simulink model "showVarLimIntegrator"  (R2023b)
settings: Solver=VariableStepAuto  StartTime=0.0  StopTime=100  RelTol=1e-3
settings Model: Creator=grouleau  LastModifiedBy=grouleau

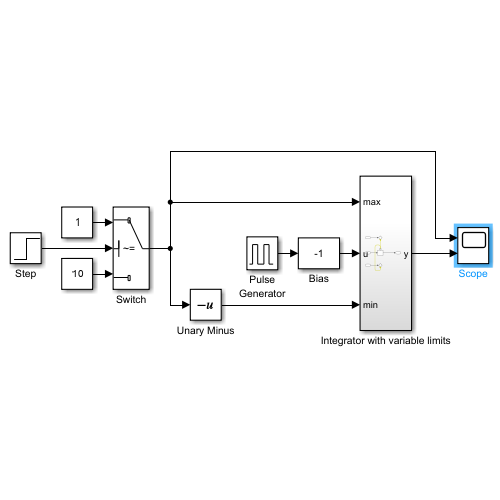
[thumbnail: Simulink's stored preview of the top-level diagram]
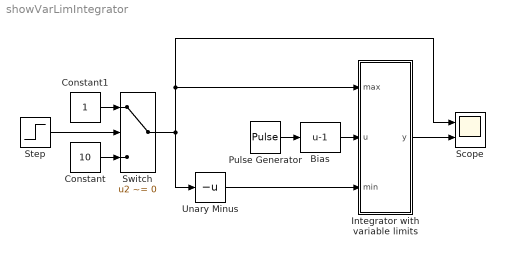
== system showVarLimIntegrator ==
  Bias : Bias  Bias=-1  SaturateOnIntegerOverflow=off
  Constant : Constant  Value=10
  Constant1 : Constant
  Integrator with variable limits : Subsystem
  Pulse Generator : DiscretePulseGenerator  PulseType=Time based  Amplitude=2  Period=10  PulseWidth=50
  Scope : Scope  NumInputPorts=2
  Step : Step  Time=50  SampleTime=0
  Switch : Switch  Criteria=u2 ~= 0  SaturateOnIntegerOverflow=off  InputSameDT=off
  Unary Minus : UnaryMinus
  wires:
  Pulse Generator/1 -> Bias/1
  Switch/1 -> Scope/1, Integrator with variable limits/1(max), Unary Minus/1
  Constant1/1 -> Switch/1
  Constant/1 -> Switch/3
  Step/1 -> Switch/2
  Unary Minus/1 -> Integrator with variable limits/3(min)
  Bias/1 -> Integrator with variable limits/2(u)
  Integrator with variable limits/1(y) -> Scope/2

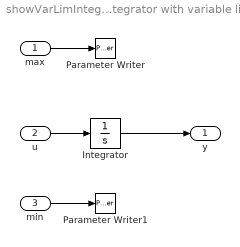
== system showVarLimIntegrator/Integrator with variable limits ==
  max : Inport
  u : Inport  Port=2
  min : Inport  Port=3
  Integrator : Integrator  LimitOutput=on
  Parameter Writer : ParameterWriter  ParameterOwnerBlock=../Integrator  ParameterName=UpperSaturationLimit  ParameterInternalName=UpperSaturationLimit
  Parameter Writer1 : ParameterWriter  ParameterOwnerBlock=../Integrator  ParameterName=LowerSaturationLimit  ParameterInternalName=LowerSaturationLimit
  y : Outport
  wires:
  max/1 -> Parameter Writer/1
  min/1 -> Parameter Writer1/1
  u/1 -> Integrator/1
  Integrator/1 -> y/1
